simulink library "generator_lib"  (Simulink 7.8)
settings: Solver=ode45  StartTime=0.0  StopTime=10.0  RelTol=1e-3
undefined symbols (not defined in the file): dfilt, DiscIntNeverNeededParam, fdesignblkfcn, gcbh, ph, Ts
libraries: simulink x91, rtio_opalrt_common x84, powerlib x51, simulink_extras x21, discretizing x14, rteventslib x14, dsparch4 x14, powerlib_extras x4
(part 1 of 10)
settings Model: Creator=re25624  LastModifiedBy=re25624

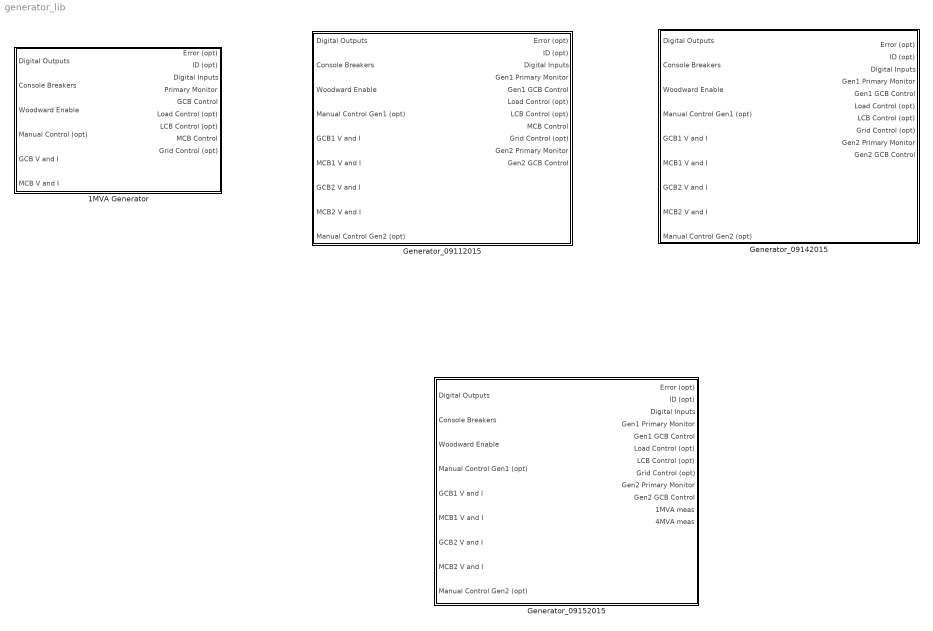
== system generator_lib ==
  1MVA Generator : Subsystem  mask{control_mode=1}
      mask prompts: control_mode "Control Mode [0 => Sim. 1 => Wood.]"
  Generator_09112015 : Subsystem
  Generator_09142015 : Subsystem
  Generator_09152015 : Subsystem  mask(Woodward and modbus controlled generators){control_mode=1}
      mask prompts: control_mode "Control Mode [0 => Sim. 1 => Wood.]"
      mask help: This block contains all the necessary logic to control two generator units (1MVA@460V and 4MVA @13.8kV) via the Woodward EasyGen controller or via Modbus commands.

== system generator_lib/1MVA Generator ==
  note: Op_Mode:
      | 0 = Relay Functions
      | 1 = Close Breaker
      | 2 = Open Breaker
  note: The woodward is set to VF mode the entire time.
  Digital Outputs : Inport
  Console Breakers : Inport  Port=2
  Woodward Enable : Inport  Port=3
  Manual Control (opt) : Inport  Port=4
  GCB V and I : Inport  Port=5
  MCB V and I : Inport  Port=6
  Bus Selector1 : BusSelector  OutputSignals=Vabc_line,Iabc
  Bus Selector5 : BusSelector  OutputSignals=Wood_DIO,Gen_bias_enable,Gen_enable,GCB,Load,LCB,Wood_MCB_enable,MCB,Grid
  Bus Selector6 : BusSelector  OutputSignals=Vabc_bus,Iabc
  Bus Selector7 : BusSelector  OutputSignals="w.w.Rotor speed  wm (pu)"
  GenSet_900kW_07232015 : Subsystem  mask(Gen-Set with simulated control modes){control_mode=control_mode}
      mask prompts: control_mode "Control Mode [0 => Sim. 1 => Wood.]"
      mask help:
      | This Gen-Set block allows the user to indicate the control mode of the generator. The available control modes are: (1) PQ, (2) PV, and (3) VF.
      | The input values to the block will be applied according to the selected control mode.
      | For example, if PQ mode is selected, the controller will only work based on P_ref and Q_ref ignoring values of other inputs to the block.
  Switch : Switch  Threshold=0.5
  Woodward Inputs : Subsystem
  Woodward Outputs : Subsystem
  A : PMIOPort  Port=1  Side=Right
  B : PMIOPort  Port=2  Side=Right
  C : PMIOPort  Port=3  Side=Right
  Error (opt) : Outport
  ID (opt) : Outport  Port=2
  Digital Inputs : Outport  Port=3
  Primary Monitor : Outport  Port=4
  GCB Control : Outport  Port=5
  Load Control (opt) : Outport  Port=6
  LCB Control (opt) : Outport  Port=7
  MCB Control : Outport  Port=8
  Grid Control (opt) : Outport  Port=9
  wires:
  Bus Selector1/2 -> Woodward Inputs/5(Mains_Current)  "<Iabc>"
  Bus Selector1/1 -> Woodward Inputs/4(Mains_Voltage)  "<Vabc_line>"
  MCB V and I/1 -> Bus Selector1/1
  Bus Selector5/9 -> Grid Control (opt)/1  "<Grid>"
  Switch/1 -> MCB Control/1
  Bus Selector5/6 -> LCB Control (opt)/1  "<LCB>"
  Bus Selector5/5 -> Load Control (opt)/1  "<Load>"
  Console Breakers/1 -> Bus Selector5/1
  Woodward Outputs/9(GCB) -> GCB Control/1
  GCB V and I/1 -> Bus Selector6/1
  Digital Outputs/1 -> Woodward Outputs/1(Digital Output)
  Woodward Outputs/10(MCB) -> Switch/1
  Bus Selector5/8 -> Switch/3  "<MCB>"
  Bus Selector5/7 -> Switch/2  "<Wood_MCB_enable>"
  Woodward Outputs/8(Fuel Enable) -> GenSet_900kW_07232015/5(Generator Enable)
  Woodward Enable/1 -> GenSet_900kW_07232015/6(Woodward Enable)
  Woodward Outputs/3(Digital Inputs) -> Digital Inputs/1
  Woodward Outputs/2(IDs) -> ID (opt)/1
  Woodward Outputs/1(Error) -> Error (opt)/1
  Bus Selector7/1 -> Woodward Inputs/1(MPU_speed)  "<Rotor speed  wm (pu)>"
  Woodward Outputs/5(Ref AVR) -> GenSet_900kW_07232015/2(Woodward Modbus Ref for AVR)
  Woodward Outputs/4(Ref Gov) -> GenSet_900kW_07232015/1(Woodward Modbus Ref for Governor)
  Bus Selector5/2 -> Woodward Outputs/3(Bias Enable)  "<Gen_bias_enable>"
  Woodward Outputs/7(AVR) -> GenSet_900kW_07232015/4(Woodward meas V)
  Woodward Outputs/6(GOV) -> GenSet_900kW_07232015/3(Woodward meas w)
  Manual Control (opt)/1 -> GenSet_900kW_07232015/7(Manual_control)
  Bus Selector5/1 -> Woodward Outputs/2(DIO Enable)  "<Wood_DIO>"
  Bus Selector6/2 -> Woodward Inputs/3(Generator_Current)  "<Iabc>"
  Bus Selector6/1 -> Woodward Inputs/2(Generator_Voltage)  "<Vabc_bus>"
  GenSet_900kW_07232015/1(gen_primary) -> Primary Monitor/1, Bus Selector7/1
  connections:
  C/RConn1 -- GenSet_900kW_07232015/RConn3
  B/RConn1 -- GenSet_900kW_07232015/RConn2
  A/RConn1 -- GenSet_900kW_07232015/RConn1

== system generator_lib/Generator_09112015 ==
  note: Ask Kendall about the output control: MCB control (8)
  note: The woodward is set to VF mode the entire time.
  note: Op_Mode:
      | 0 = Relay Functions
      | 1 = Close Breaker
      | 2 = Open Breaker
  note: Gen1: 1MVA at 460V
      | Gen2: 4MVA at 13kV
  Digital Outputs : Inport
  Console Breakers : Inport  Port=2
  Woodward Enable : Inport  Port=3
  Manual Control Gen1 (opt) : Inport  Port=4
  GCB1 V and I : Inport  Port=5
  MCB1 V and I : Inport  Port=6
  GCB2 V and I : Inport  Port=7
  MCB2 V and I : Inport  Port=8
  Manual Control Gen2 (opt) : Inport  Port=9
  Bus Selector : BusSelector  OutputSignals=Gen1 Ref GOV,Gen1 Ref AVR,Gen1 Gov,Gen1 AVR
  Bus Selector1 : BusSelector  OutputSignals=Vabc_bus,Iabc
  Bus Selector2 : BusSelector  OutputSignals="w.w.Rotor speed  wm (pu)"
  Bus Selector3 : BusSelector  OutputSignals=Vabc_line,Iabc
  Bus Selector4 : BusSelector  OutputSignals=Vabc_bus,Iabc
  Bus Selector5 : BusSelector  OutputSignals=Wood_DIO,Gen_bias_enable,Gen2_enable,Gen2_GCB,Load,LCB,Wood_MCB_enable,MCB,Grid
  Bus Selector6 : BusSelector  OutputSignals=Vabc_line,Iabc
  Bus Selector7 : BusSelector  OutputSignals="w.w.Rotor speed  wm (pu)"
  Bus Selector8 : BusSelector  OutputSignals=Gen2 Ref GOV,Gen2 Ref AVR,Gen2 GOV,Gen2 AVR
  GenSet_1MVA_09082015 : Subsystem  mask(Gen-Set with simulated control modes){control_mode=1}
      mask prompts: control_mode "Control Mode [0 => Sim. 1 => Wood.]"
      mask help:
      | This Gen-Set block allows the user to indicate the control mode of the generator. The available control modes are: (1) PQ, (2) PV, and (3) VF.
      | The input values to the block will be applied according to the selected control mode.
      | For example, if PQ mode is selected, the controller will only work based on P_ref and Q_ref ignoring values of other inputs to the block.
  GenSet_4MVA_copy1mva : Subsystem  mask(Gen-Set with simulated control modes){control_mode=1}
      mask prompts: control_mode "Control Mode [0 => Sim. 1 => Wood.]"
      mask help:
      | This Gen-Set block allows the user to indicate the control mode of the generator. The available control modes are: (1) PQ, (2) PV, and (3) VF.
      | The input values to the block will be applied according to the selected control mode.
      | For example, if PQ mode is selected, the controller will only work based on P_ref and Q_ref ignoring values of other inputs to the block.
  Switch : Switch  Threshold=0.5
  Woodward Inputs : Subsystem
  Woodward Outputs : Subsystem
  Gen2 A : PMIOPort  Port=1  Side=Right
  Gen2 B : PMIOPort  Port=2  Side=Right
  Gen2 C : PMIOPort  Port=3  Side=Right
  Gen1 A : PMIOPort  Port=4  Side=Right
  Gen1 B : PMIOPort  Port=5  Side=Right
  Gen1 C : PMIOPort  Port=6  Side=Right
  Error (opt) : Outport
  ID (opt) : Outport  Port=2
  Digital Inputs : Outport  Port=3
  Gen1 Primary Monitor : Outport  Port=4
  Gen1 GCB Control : Outport  Port=5
  Load Control (opt) : Outport  Port=6
  LCB Control (opt) : Outport  Port=7
  MCB Control : Outport  Port=8
  Grid Control (opt) : Outport  Port=9
  Gen2 Primary Monitor : Outport  Port=10
  Gen2 GCB Control : Outport  Port=11
  wires:
  GenSet_1MVA_09082015/1(gen_primary) -> Bus Selector7/1, Gen1 Primary Monitor/1
  Bus Selector6/1 -> Woodward Inputs/2(Generator1_Voltage)  "<Vabc_line>"
  Bus Selector6/2 -> Woodward Inputs/3(Generator1_Current)  "<Iabc>"
  Bus Selector5/1 -> Woodward Outputs/2(DIO Enable)  "<Wood_DIO>"
  Manual Control Gen1 (opt)/1 -> GenSet_1MVA_09082015/7(Manual_control)
  Bus Selector5/2 -> Woodward Outputs/3(Bias Enable)  "<Gen_bias_enable>"
  Bus Selector7/1 -> Woodward Inputs/1(MPU1_speed)  "<Rotor speed  wm (pu)>"
  Woodward Outputs/1(Error) -> Error (opt)/1
  Woodward Outputs/2(IDs) -> ID (opt)/1
  Woodward Outputs/3(Digital Inputs) -> Digital Inputs/1
  Woodward Enable/1 -> GenSet_1MVA_09082015/6(Woodward Enable), GenSet_4MVA_copy1mva/6(Woodward Enable)
  Woodward Outputs/6(Gen1 Fuel Enable) -> GenSet_1MVA_09082015/5(Generator Enable)
  Bus Selector5/7 -> Switch/2  "<Wood_MCB_enable>"
  Bus Selector5/8 -> Switch/3  "<MCB>"
  Woodward Outputs/8(Gen1 MCB) -> Switch/1
  Digital Outputs/1 -> Woodward Outputs/1(Digital Output)
  GCB1 V and I/1 -> Bus Selector6/1
  Woodward Outputs/7(Gen1 GCB) -> Gen1 GCB Control/1
  Console Breakers/1 -> Bus Selector5/1
  Bus Selector5/5 -> Load Control (opt)/1  "<Load>"
  Bus Selector5/6 -> LCB Control (opt)/1  "<LCB>"
  Switch/1 -> MCB Control/1
  Bus Selector5/9 -> Grid Control (opt)/1  "<Grid>"
  MCB1 V and I/1 -> Bus Selector1/1
  Bus Selector1/1 -> Woodward Inputs/4(Mains1_Voltage)  "<Vabc_bus>"
  Bus Selector1/2 -> Woodward Inputs/5(Mains1_Current)  "<Iabc>"
  GCB2 V and I/1 -> Bus Selector3/1
  MCB2 V and I/1 -> Bus Selector4/1
  GenSet_4MVA_copy1mva/1(gen_primary) -> Gen2 Primary Monitor/1, Bus Selector2/1
  Bus Selector2/1 -> Woodward Inputs/6(MPU2_speed)  "<Rotor speed  wm (pu)>"
  Bus Selector3/1 -> Woodward Inputs/7(Generator2_Voltage)  "<Vabc_line>"
  Bus Selector3/2 -> Woodward Inputs/8(Generator2_Current)  "<Iabc>"
  Bus Selector4/1 -> Woodward Inputs/9(Mains2_Voltage)  "<Vabc_bus>"
  Bus Selector4/2 -> Woodward Inputs/10(Mains2_Current)  "<Iabc>"
  Woodward Outputs/4(Gen1 Gov and AVR) -> Bus Selector/1
  Bus Selector/1 -> GenSet_1MVA_09082015/1(Woodward Modbus Ref for Governor)  "<Gen1 Ref GOV>"
  Bus Selector/2 -> GenSet_1MVA_09082015/2(Woodward Modbus Ref for AVR)  "<Gen1 Ref AVR>"
  Bus Selector/3 -> GenSet_1MVA_09082015/3(Woodward meas w)  "<Gen1 Gov>"
  Bus Selector/4 -> GenSet_1MVA_09082015/4(Woodward meas V)  "<Gen1 AVR>"
  Woodward Outputs/5(Gen2 Gov and AVR) -> Bus Selector8/1
  Bus Selector8/1 -> GenSet_4MVA_copy1mva/1(Woodward Modbus Ref for Governor)  "<Gen2 Ref GOV>"
  Bus Selector8/2 -> GenSet_4MVA_copy1mva/2(Woodward Modbus Ref for AVR)  "<Gen2 Ref AVR>"
  Bus Selector8/3 -> GenSet_4MVA_copy1mva/3(Woodward meas w)  "<Gen2 GOV>"
  Bus Selector8/4 -> GenSet_4MVA_copy1mva/4(Woodward meas V)  "<Gen2 AVR>"
  Manual Control Gen2 (opt)/1 -> GenSet_4MVA_copy1mva/7(Manual_control)
  Woodward Outputs/9(Gen2 Fuel Enable) -> GenSet_4MVA_copy1mva/5(Generator Enable)
  Woodward Outputs/10(Gen2 GCB) -> Gen2 GCB Control/1
  connections:
  Gen1 A/RConn1 -- GenSet_1MVA_09082015/RConn1
  Gen1 B/RConn1 -- GenSet_1MVA_09082015/RConn2
  Gen1 C/RConn1 -- GenSet_1MVA_09082015/RConn3
  GenSet_4MVA_copy1mva/RConn1 -- Gen2 A/RConn1
  GenSet_4MVA_copy1mva/RConn2 -- Gen2 B/RConn1
  GenSet_4MVA_copy1mva/RConn3 -- Gen2 C/RConn1

== system generator_lib/Generator_09142015 ==
  note: Gen1: 1MVA generator
      | Gen2: 4MVA generator
  note: Op_Mode:
      | 0 = Relay Functions
      | 1 = Close Breaker
      | 2 = Open Breaker
  note: The woodward is set to VF mode the entire time.
  Digital Outputs : Inport
  Console Breakers : Inport  Port=2
  Woodward Enable : Inport  Port=3
  Manual Control Gen1 (opt) : Inport  Port=4
  GCB1 V and I : Inport  Port=5
  MCB1 V and I : Inport  Port=6
  GCB2 V and I : Inport  Port=7
  MCB2 V and I : Inport  Port=8
  Manual Control Gen2 (opt) : Inport  Port=9
  Add : Sum  Inputs=+-
  Bus Selector : BusSelector  OutputSignals=Gen1 Ref GOV,Gen1 Ref AVR,Gen1 Gov,Gen1 AVR
  Bus Selector1 : BusSelector  OutputSignals=Vabc_line,Iabc
  Bus Selector2 : BusSelector  OutputSignals="w.w.Rotor speed  wm (pu)"
  Bus Selector3 : BusSelector  OutputSignals=Vabc_bus,Iabc
  Bus Selector4 : BusSelector  OutputSignals=Vabc_line,Iabc
  Bus Selector5 : BusSelector  OutputSignals=Wood_DIO,Gen_bias_enable,Gen2_enable,Gen2_GCB,Load,LCB,Wood_MCB_enable,MCB,Grid
  Bus Selector6 : BusSelector  OutputSignals=Vabc_bus,Iabc
  Bus Selector7 : BusSelector  OutputSignals="w.w.Rotor speed  wm (pu)"
  Bus Selector8 : BusSelector  OutputSignals=Gen2 Ref GOV,Gen2 Ref AVR,Gen2 GOV,Gen2 AVR
  Constant : Constant  Value=0.01
  GenSet_1MVA_09082015 : Subsystem  mask(Gen-Set with simulated control modes){control_mode=1}
      mask prompts: control_mode "Control Mode [0 => Sim. 1 => Wood.]"
      mask help:
      | This Gen-Set block allows the user to indicate the control mode of the generator. The available control modes are: (1) PQ, (2) PV, and (3) VF.
      | The input values to the block will be applied according to the selected control mode.
      | For example, if PQ mode is selected, the controller will only work based on P_ref and Q_ref ignoring values of other inputs to the block.
  GenSet_4MVA_09142015 : Subsystem  mask(Gen-Set with simulated control modes){control_mode=1}
      mask prompts: control_mode "Control Mode [0 => Sim. 1 => Wood.]"
      mask help:
      | This Gen-Set block allows the user to indicate the control mode of the generator. The available control modes are: (1) PQ, (2) PV, and (3) VF.
      | The input values to the block will be applied according to the selected control mode.
      | For example, if PQ mode is selected, the controller will only work based on P_ref and Q_ref ignoring values of other inputs to the block.
  Woodward Inputs : Subsystem
  Woodward Outputs : Subsystem
  Gen2 A : PMIOPort  Port=1  Side=Right
  Gen2 B : PMIOPort  Port=2  Side=Right
  Gen2 C : PMIOPort  Port=3  Side=Right
  Gen1 A : PMIOPort  Port=4  Side=Right
  Gen1 B : PMIOPort  Port=5  Side=Right
  Gen1 C : PMIOPort  Port=6  Side=Right
  Error (opt) : Outport
  ID (opt) : Outport  Port=2
  Digital Inputs : Outport  Port=3
  Gen1 Primary Monitor : Outport  Port=4
  Gen1 GCB Control : Outport  Port=5
  Load Control (opt) : Outport  Port=6
  LCB Control (opt) : Outport  Port=7
  Grid Control (opt) : Outport  Port=8
  Gen2 Primary Monitor : Outport  Port=9
  Gen2 GCB Control : Outport  Port=10
  wires:
  Constant/1 -> Add/2
  Add/1 -> Woodward Inputs/6(MPU2_speed)
  Woodward Outputs/10(Gen2 GCB) -> Gen2 GCB Control/1
  Woodward Outputs/9(Gen2 Fuel Enable) -> GenSet_4MVA_09142015/5(Generator Enable)
  Manual Control Gen2 (opt)/1 -> GenSet_4MVA_09142015/7(Manual_control)
  Bus Selector8/4 -> GenSet_4MVA_09142015/4(Woodward meas V)  "<Gen2 AVR>"
  Bus Selector8/3 -> GenSet_4MVA_09142015/3(Woodward meas w)  "<Gen2 GOV>"
  Bus Selector8/2 -> GenSet_4MVA_09142015/2(Woodward Modbus Ref for AVR)  "<Gen2 Ref AVR>"
  Bus Selector8/1 -> GenSet_4MVA_09142015/1(Woodward Modbus Ref for Governor)  "<Gen2 Ref GOV>"
  Woodward Outputs/5(Gen2 Gov and AVR) -> Bus Selector8/1
  Bus Selector/4 -> GenSet_1MVA_09082015/4(Woodward meas V)  "<Gen1 AVR>"
  Bus Selector/3 -> GenSet_1MVA_09082015/3(Woodward meas w)  "<Gen1 Gov>"
  Bus Selector/2 -> GenSet_1MVA_09082015/2(Woodward Modbus Ref for AVR)  "<Gen1 Ref AVR>"
  Bus Selector/1 -> GenSet_1MVA_09082015/1(Woodward Modbus Ref for Governor)  "<Gen1 Ref GOV>"
  Woodward Outputs/4(Gen1 Gov and AVR) -> Bus Selector/1
  Bus Selector4/2 -> Woodward Inputs/10(Mains2_Current)  "<Iabc>"
  Bus Selector4/1 -> Woodward Inputs/9(Mains2_Voltage)  "<Vabc_line>"
  Bus Selector3/2 -> Woodward Inputs/8(Generator2_Current)  "<Iabc>"
  Bus Selector3/1 -> Woodward Inputs/7(Generator2_Voltage)  "<Vabc_bus>"
  Bus Selector2/1 -> Add/1  "<Rotor speed  wm (pu)>"
  GenSet_4MVA_09142015/1(gen_primary) -> Bus Selector2/1, Gen2 Primary Monitor/1
  MCB2 V and I/1 -> Bus Selector4/1
  GCB2 V and I/1 -> Bus Selector3/1
  Bus Selector1/2 -> Woodward Inputs/5(Mains1_Current)  "<Iabc>"
  Bus Selector1/1 -> Woodward Inputs/4(Mains1_Voltage)  "<Vabc_line>"
  MCB1 V and I/1 -> Bus Selector1/1
  Bus Selector5/9 -> Grid Control (opt)/1  "<Grid>"
  Bus Selector5/6 -> LCB Control (opt)/1  "<LCB>"
  Bus Selector5/5 -> Load Control (opt)/1  "<Load>"
  Console Breakers/1 -> Bus Selector5/1
  Woodward Outputs/7(Gen1 GCB) -> Gen1 GCB Control/1
  GCB1 V and I/1 -> Bus Selector6/1
  Digital Outputs/1 -> Woodward Outputs/1(Digital Output)
  Woodward Outputs/6(Gen1 Fuel Enable) -> GenSet_1MVA_09082015/5(Generator Enable)
  Woodward Enable/1 -> GenSet_4MVA_09142015/6(Woodward Enable), GenSet_1MVA_09082015/6(Woodward Enable)
  Woodward Outputs/3(Digital Inputs) -> Digital Inputs/1
  Woodward Outputs/2(IDs) -> ID (opt)/1
  Woodward Outputs/1(Error) -> Error (opt)/1
  Bus Selector7/1 -> Woodward Inputs/1(MPU1_speed)  "<Rotor speed  wm (pu)>"
  Bus Selector5/2 -> Woodward Outputs/3(Bias Enable)  "<Gen_bias_enable>"
  Manual Control Gen1 (opt)/1 -> GenSet_1MVA_09082015/7(Manual_control)
  Bus Selector5/1 -> Woodward Outputs/2(DIO Enable)  "<Wood_DIO>"
  Bus Selector6/2 -> Woodward Inputs/3(Generator1_Current)  "<Iabc>"
  Bus Selector6/1 -> Woodward Inputs/2(Generator1_Voltage)  "<Vabc_bus>"
  GenSet_1MVA_09082015/1(gen_primary) -> Gen1 Primary Monitor/1, Bus Selector7/1
  connections:
  GenSet_4MVA_09142015/RConn3 -- Gen2 C/RConn1
  GenSet_4MVA_09142015/RConn2 -- Gen2 B/RConn1
  GenSet_4MVA_09142015/RConn1 -- Gen2 A/RConn1
  Gen1 C/RConn1 -- GenSet_1MVA_09082015/RConn3
  Gen1 B/RConn1 -- GenSet_1MVA_09082015/RConn2
  Gen1 A/RConn1 -- GenSet_1MVA_09082015/RConn1

== system generator_lib/Generator_09152015 ==
  note: Gen1: 1MVA generator
      | Gen2: 4MVA generator
  note: Op_Mode:
      | 0 = Relay Functions
      | 1 = Close Breaker
      | 2 = Open Breaker
  note: The woodward is set to VF mode the entire time.
  note: When used in the system to be simulated,
      | this model most be disabled from the library or the I/Os will have an error
  Digital Outputs : Inport
  Console Breakers : Inport  Port=2
  Woodward Enable : Inport  Port=3
  Manual Control Gen1 (opt) : Inport  Port=4
  GCB1 V and I : Inport  Port=5
  MCB1 V and I : Inport  Port=6
  GCB2 V and I : Inport  Port=7
  MCB2 V and I : Inport  Port=8
  Manual Control Gen2 (opt) : Inport  Port=9
  Add : Sum  Inputs=+-
  Bus Selector : BusSelector  OutputSignals=Gen1 Ref GOV,Gen1 Ref AVR,Gen1 Gov,Gen1 AVR
  Bus Selector1 : BusSelector  OutputSignals=Vabc_line,Iabc
  Bus Selector2 : BusSelector  OutputSignals="w.w.Rotor speed  wm (pu)"
  Bus Selector3 : BusSelector  OutputSignals=Vabc_bus,Iabc
  Bus Selector4 : BusSelector  OutputSignals=Vabc_line,Iabc
  Bus Selector5 : BusSelector  OutputSignals=Wood_DIO,Gen_bias_enable,Gen2_enable,Gen2_GCB,Load,LCB,Wood_MCB_enable,MCB,Grid
  Bus Selector6 : BusSelector  OutputSignals=Vabc_bus,Iabc
  Bus Selector7 : BusSelector  OutputSignals="w.w.Rotor speed  wm (pu)"
  Bus Selector8 : BusSelector  OutputSignals=Gen2 Ref GOV,Gen2 Ref AVR,Gen2 GOV,Gen2 AVR
  Constant : Constant  Value=0.01
  GenSet_1MVA_09082015 : Subsystem  mask(Gen-Set with simulated control modes){control_mode=control_mode}
      mask prompts: control_mode "Control Mode [0 => Sim. 1 => Wood.]"
      mask help:
      | This Gen-Set block allows the user to indicate the control mode of the generator. The available control modes are: (1) PQ, (2) PV, and (3) VF.
      | The input values to the block will be applied according to the selected control mode.
      | For example, if PQ mode is selected, the controller will only work based on P_ref and Q_ref ignoring values of other inputs to the block.
  GenSet_4MVA_09142015 : Subsystem  mask(Gen-Set with simulated control modes){control_mode=control_mode}
      mask prompts: control_mode "Control Mode [0 => Sim. 1 => Wood.]"
      mask help:
      | This Gen-Set block allows the user to indicate the control mode of the generator. The available control modes are: (1) PQ, (2) PV, and (3) VF.
      | The input values to the block will be applied according to the selected control mode.
      | For example, if PQ mode is selected, the controller will only work based on P_ref and Q_ref ignoring values of other inputs to the block.
  Woodward Inputs : Subsystem
  Woodward Outputs : Subsystem
  Gen2 A : PMIOPort  Port=1  Side=Right
  Gen2 B : PMIOPort  Port=2  Side=Right
  Gen2 C : PMIOPort  Port=3  Side=Right
  Gen1 A : PMIOPort  Port=4  Side=Right
  Gen1 B : PMIOPort  Port=5  Side=Right
  Gen1 C : PMIOPort  Port=6  Side=Right
  Error (opt) : Outport
  ID (opt) : Outport  Port=2
  Digital Inputs : Outport  Port=3
  Gen1 Primary Monitor : Outport  Port=4
  Gen1 GCB Control : Outport  Port=5
  Load Control (opt) : Outport  Port=6
  LCB Control (opt) : Outport  Port=7
  Grid Control (opt) : Outport  Port=8
  Gen2 Primary Monitor : Outport  Port=9
  Gen2 GCB Control : Outport  Port=10
  1MVA meas : Outport  Port=11
  4MVA meas : Outport  Port=12
  wires:
  GenSet_4MVA_09142015/2(gen_output) -> 4MVA meas/1
  GenSet_1MVA_09082015/2(gen_output) -> 1MVA meas/1
  Constant/1 -> Add/2
  Add/1 -> Woodward Inputs/6(MPU2_speed)
  Woodward Outputs/10(Gen2 GCB) -> Gen2 GCB Control/1
  Woodward Outputs/9(Gen2 Fuel Enable) -> GenSet_4MVA_09142015/5(Generator Enable)
  Manual Control Gen2 (opt)/1 -> GenSet_4MVA_09142015/7(Manual_control)
  Bus Selector8/4 -> GenSet_4MVA_09142015/4(Woodward meas V)  "<Gen2 AVR>"
  Bus Selector8/3 -> GenSet_4MVA_09142015/3(Woodward meas w)  "<Gen2 GOV>"
  Bus Selector8/2 -> GenSet_4MVA_09142015/2(Woodward Modbus Ref for AVR)  "<Gen2 Ref AVR>"
  Bus Selector8/1 -> GenSet_4MVA_09142015/1(Woodward Modbus Ref for Governor)  "<Gen2 Ref GOV>"
  Woodward Outputs/5(Gen2 Gov and AVR) -> Bus Selector8/1
  Bus Selector/4 -> GenSet_1MVA_09082015/4(Woodward meas V)  "<Gen1 AVR>"
  Bus Selector/3 -> GenSet_1MVA_09082015/3(Woodward meas w)  "<Gen1 Gov>"
  Bus Selector/2 -> GenSet_1MVA_09082015/2(Woodward Modbus Ref for AVR)  "<Gen1 Ref AVR>"
  Bus Selector/1 -> GenSet_1MVA_09082015/1(Woodward Modbus Ref for Governor)  "<Gen1 Ref GOV>"
  Woodward Outputs/4(Gen1 Gov and AVR) -> Bus Selector/1
  Bus Selector4/2 -> Woodward Inputs/10(Mains2_Current)  "<Iabc>"
  Bus Selector4/1 -> Woodward Inputs/9(Mains2_Voltage)  "<Vabc_line>"
  Bus Selector3/2 -> Woodward Inputs/8(Generator2_Current)  "<Iabc>"
  Bus Selector3/1 -> Woodward Inputs/7(Generator2_Voltage)  "<Vabc_bus>"
  Bus Selector2/1 -> Add/1  "<Rotor speed  wm (pu)>"
  GenSet_4MVA_09142015/1(gen_primary) -> Bus Selector2/1, Gen2 Primary Monitor/1
  MCB2 V and I/1 -> Bus Selector4/1
  GCB2 V and I/1 -> Bus Selector3/1
  Bus Selector1/2 -> Woodward Inputs/5(Mains1_Current)  "<Iabc>"
  Bus Selector1/1 -> Woodward Inputs/4(Mains1_Voltage)  "<Vabc_line>"
  MCB1 V and I/1 -> Bus Selector1/1
  Bus Selector5/9 -> Grid Control (opt)/1  "<Grid>"
  Bus Selector5/6 -> LCB Control (opt)/1  "<LCB>"
  Bus Selector5/5 -> Load Control (opt)/1  "<Load>"
  Console Breakers/1 -> Bus Selector5/1
  Woodward Outputs/7(Gen1 GCB) -> Gen1 GCB Control/1
  GCB1 V and I/1 -> Bus Selector6/1
  Digital Outputs/1 -> Woodward Outputs/1(Digital Output)
  Woodward Outputs/6(Gen1 Fuel Enable) -> GenSet_1MVA_09082015/5(Generator Enable)
  Woodward Enable/1 -> GenSet_4MVA_09142015/6(Woodward Enable), GenSet_1MVA_09082015/6(Woodward Enable)
  Woodward Outputs/3(Digital Inputs) -> Digital Inputs/1
  Woodward Outputs/2(IDs) -> ID (opt)/1
  Woodward Outputs/1(Error) -> Error (opt)/1
  Bus Selector7/1 -> Woodward Inputs/1(MPU1_speed)  "<Rotor speed  wm (pu)>"
  Bus Selector5/2 -> Woodward Outputs/3(Bias Enable)  "<Gen_bias_enable>"
  Manual Control Gen1 (opt)/1 -> GenSet_1MVA_09082015/7(Manual_control)
  Bus Selector5/1 -> Woodward Outputs/2(DIO Enable)  "<Wood_DIO>"
  Bus Selector6/2 -> Woodward Inputs/3(Generator1_Current)  "<Iabc>"
  Bus Selector6/1 -> Woodward Inputs/2(Generator1_Voltage)  "<Vabc_bus>"
  GenSet_1MVA_09082015/1(gen_primary) -> Gen1 Primary Monitor/1, Bus Selector7/1
  connections:
  GenSet_4MVA_09142015/RConn3 -- Gen2 C/RConn1
  GenSet_4MVA_09142015/RConn2 -- Gen2 B/RConn1
  GenSet_4MVA_09142015/RConn1 -- Gen2 A/RConn1
  Gen1 C/RConn1 -- GenSet_1MVA_09082015/RConn3
  Gen1 B/RConn1 -- GenSet_1MVA_09082015/RConn2
  Gen1 A/RConn1 -- GenSet_1MVA_09082015/RConn1

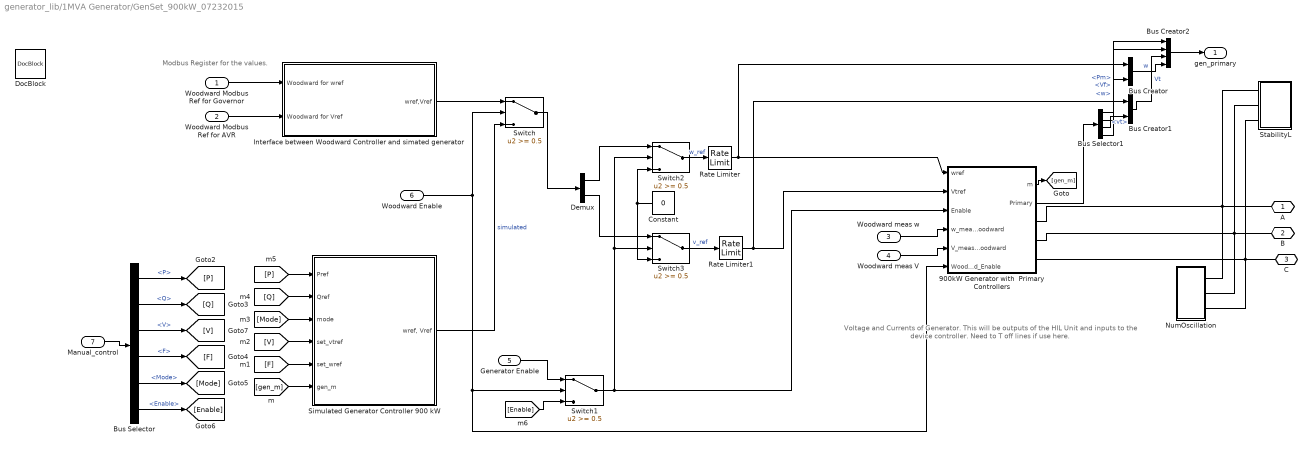
== system generator_lib/1MVA Generator/GenSet_900kW_07232015 ==
  note: Voltage and Currents of Generator.
      | This will be outputs of the HIL Unit
      | and inputs to the device controller.
      | Need to T off lines if use here.
  note: Modbus Register for the values.
  Woodward Modbus Ref for Governor : Inport
  Woodward Modbus Ref for AVR : Inport  Port=2
  Woodward meas w : Inport  Port=3
  Woodward meas V : Inport  Port=4
  Generator Enable : Inport  Port=5
  Woodward Enable : Inport  Port=6
  Manual_control : Inport  Port=7
  900kW Generator with  Primary Controllers : Subsystem
  Bus Creator : BusCreator  Inputs=2
  Bus Creator1 : BusCreator  Inputs=2
  Bus Creator2 : BusCreator
  Bus Selector : BusSelector  OutputSignals=P,Q,V,F,Mode,Enable
  Bus Selector1 : BusSelector  OutputSignals=Pm,Vf,vt,w
  Constant : Constant  Value=0
  Demux : Demux  Outputs=2
  DocBlock : simulink/Model-Wide Utilities/DocBlock  DocumentType=Text
  Interface between Woodward Controller and simated generator : Subsystem
  NumOscillation : Subsystem
  Rate Limiter : RateLimiter  RisingSlewLimit=0.5  FallingSlewLimit=-0.5  SampleTimeMode=inherited
  Rate Limiter1 : RateLimiter  RisingSlewLimit=0.5  FallingSlewLimit=-0.5  SampleTimeMode=inherited
  Simulated Generator Controller 900 kW : Subsystem
  StabilityL : Subsystem  mask{v=460, kVA=50, pf=1}
  Switch{,1..3} (4 alike) : Switch  Threshold=0.5
  A : PMIOPort  Port=1  Side=Right
  B : PMIOPort  Port=2  Side=Right
  C : PMIOPort  Port=3  Side=Right
  gen_primary : Outport
  wires:
  Woodward Enable/1 -> 900kW Generator with  Primary Controllers/6(Woodward_Enable), Switch1/2, Switch/2
  Rate Limiter1/1 -> Bus Creator1/1, 900kW Generator with  Primary Controllers/2(Vtref)
  Rate Limiter/1 -> Bus Creator/1, 900kW Generator with  Primary Controllers/1(wref)
  Bus Creator2/1 -> gen_primary/1
  Bus Creator/1 -> Bus Creator2/4  "w"
  Bus Creator1/1 -> Bus Creator2/3  "Vt"
  Bus Selector1/1 -> Bus Creator2/1  "<Pm>"
  Bus Selector1/2 -> Bus Creator2/2  "<Vf>"
  Bus Selector1/4 -> Bus Creator/2  "<w>"
  Bus Selector1/3 -> Bus Creator1/2  "<vt>"
  Switch3/1 -> Rate Limiter1/1  "v_ref"
  Constant/1 -> Switch2/3, Switch3/3
  Demux/2 -> Switch3/1
  Demux/1 -> Switch2/1
  Switch2/1 -> Rate Limiter/1  "w_ref"
  Switch1/1 -> Switch3/2, Switch2/2, 900kW Generator with  Primary Controllers/3(Enable)
  [Enable] -> Switch1/3
  Generator Enable/1 -> Switch1/1
  900kW Generator with  Primary Controllers/2(Primary) -> Bus Selector1/1
  Bus Selector/6 -> [Enable]  "<Enable>"
  Woodward meas V/1 -> 900kW Generator with  Primary Controllers/5(V_meas_Woodward)
  Woodward meas w/1 -> 900kW Generator with  Primary Controllers/4(w_meas_Woodward)
  Woodward Modbus Ref for AVR/1 -> Interface between Woodward Controller and simated generator/2(Woodward for Vref)
  Woodward Modbus Ref for Governor/1 -> Interface between Woodward Controller and simated generator/1(Woodward for wref)
  Switch/1 -> Demux/1
  Interface between Woodward Controller and simated generator/1(wref,Vref) -> Switch/1
  900kW Generator with  Primary Controllers/1(m) -> [gen_m]
  Simulated Generator Controller 900 kW/1("wref, Vref") -> Switch/3  "simulated"
  Manual_control/1 -> Bus Selector/1
  Bus Selector/1 -> [P]  "<P>"
  Bus Selector/2 -> [Q]  "<Q>"
  Bus Selector/3 -> [V]  "<V>"
  Bus Selector/4 -> [F]  "<F>"
  Bus Selector/5 -> [Mode]  "<Mode>"
  [gen_m] -> Simulated Generator Controller 900 kW/6(gen_m)
  [P] -> Simulated Generator Controller 900 kW/1(Pref)
  [Q] -> Simulated Generator Controller 900 kW/2(Qref)
  [Mode] -> Simulated Generator Controller 900 kW/3(mode)
  [V] -> Simulated Generator Controller 900 kW/4(set_vtref)
  [F] -> Simulated Generator Controller 900 kW/5(set_wref)
  connections:
  NumOscillation/LConn3 -- 900kW Generator with  Primary Controllers/RConn3 -- C/RConn1 -- StabilityL/LConn3
  NumOscillation/LConn2 -- B/RConn1 -- 900kW Generator with  Primary Controllers/RConn2 -- StabilityL/LConn2
  NumOscillation/LConn1 -- 900kW Generator with  Primary Controllers/RConn1 -- A/RConn1 -- StabilityL/LConn1

== system generator_lib/1MVA Generator/Woodward Inputs ==
  note: Wood 3.5MW 3/P
      | Mains Voltage
  note: Wood 3.5MW 3/P
      | Gen. Voltage
  note: Wood 3.5MW MPU
  note: There will need to be a
      | new scaling factor to use
      | the current cards (0-1A)
  note: GR1 A AOUT (CH00-15)
  note: For 120 => 12Vout / 170Vpk
      | For 480 => 12Vout / 391Vpk
      | For 13.8kv => 12Vout / 11268Vpk
  note: 6Vout / ( 900,000W / 391 Vpk)
  MPU_speed : Inport
  Generator_Voltage : Inport  Port=2
  Generator_Current : Inport  Port=3
  Mains_Voltage : Inport  Port=4
  Mains_Current : Inport  Port=5
  AnalogOut : rtio_opalrt_common/AnalogOut  CtrlName='OpCtrl'  portNb=1  FcnNos=Slot 1 Module A Subsection 1  size=16  maxcount=-2  count=8  numchan=8  israngeinput=off  voltagerange=[-16 ... 16]  slot=0  side=0  mismatch=0  slotside=Slot_1_Module_A
      settings: AttributesFormatString=%<CtrlName>
  AnalogOut1 : rtio_opalrt_common/AnalogOut  CtrlName='OpCtrl'  portNb=2  FcnNos=Slot 1 Module A Subsection 2  size=16  maxcount=-2  count=8  numchan=8  israngeinput=off  voltagerange=[-16 ... 16]  slot=0  side=0  mismatch=0  slotside=Slot_1_Module_A
      settings: AttributesFormatString=%<CtrlName>
  AnalogOut2 : rtio_opalrt_common/AnalogOut  CtrlName='OpCtrl'  portNb=3  FcnNos=Slot 2 Module A Subsection 1  size=16  maxcount=-2  count=8  numchan=8  israngeinput=off  voltagerange=[-16 ... 16]  slot=1  side=0  mismatch=0  slotside=Slot_2_Module_A
      settings: AttributesFormatString=%<CtrlName>
  AnalogOut3 : rtio_opalrt_common/AnalogOut  CtrlName='OpCtrl'  portNb=4  FcnNos=Slot 2 Module A Subsection 2  size=16  maxcount=-2  count=8  numchan=8  israngeinput=off  voltagerange=[-16 ... 16]  slot=1  side=0  mismatch=0  slotside=Slot_2_Module_A
      settings: AttributesFormatString=%<CtrlName>
  Demux : Demux  Outputs=2
  Demux{1..5,7} (6 alike) : Demux  Outputs=3
  Demux6 : Demux  Outputs=2
  Gain : Gain  Gain=15/391
  Gain1 : Gain  Gain=15/11268
  Gain2 : Gain  Gain=15/(900000/391)
  Gain3 : Gain  Gain=15/(900000/11268)
  Mux{,1,3..4} (4 alike) : Mux  Inputs=8
  Mux2 : Mux  Inputs=2
  Mux5 : Mux  Inputs=2
  Speed_System : Subsystem
  Terminator{,1..3} (4 alike) : Terminator
  wires:
  Demux7/1 -> Mux3/1
  Gain3/1 -> Demux7/1
  Mains_Current/1 -> Gain3/1
  Demux3/3 -> Mux3/4
  Demux3/2 -> Mux3/3
  Demux3/1 -> Mux3/2
  Gain2/1 -> Demux3/1
  AnalogOut2/1 -> Terminator2/1
  AnalogOut3/1 -> Terminator3/1
  Demux6/1 -> AnalogOut2/1
  Demux6/2 -> AnalogOut3/1
  Mux3/1 -> Mux5/1
  Mux4/1 -> Mux5/2
  Mux5/1 -> Demux6/1
  Demux5/3 -> Mux1/4
  Demux5/2 -> Mux1/3
  Demux5/1 -> Mux1/2
  Demux4/3 -> Mux1/1
  Demux4/2 -> Mux/8
  Demux4/1 -> Mux/7
  Speed_System/1(Out1) -> Mux1/5
  Demux2/3 -> Mux/6
  Demux2/2 -> Mux/5
  Demux2/1 -> Mux/4
  Demux1/3 -> Mux/3
  Demux1/2 -> Mux/2
  Demux1/1 -> Mux/1
  AnalogOut/1 -> Terminator/1
  AnalogOut1/1 -> Terminator1/1
  Demux/1 -> AnalogOut/1
  Demux/2 -> AnalogOut1/1
  Generator_Voltage/1 -> Gain/1
  Mux/1 -> Mux2/1
  Mux1/1 -> Mux2/2
  Mux2/1 -> Demux/1
  Mains_Voltage/1 -> Gain1/1
  Gain/1 -> Demux1/1
  Gain1/1 -> Demux2/1
  Generator_Current/1 -> Gain2/1
  MPU_speed/1 -> Speed_System/1(In1)

== system generator_lib/1MVA Generator/Woodward Outputs ==
  Digital Output : Inport
  DIO Enable : Inport  Port=2
  Bias Enable : Inport  Port=3
  Bus Creator1 : BusCreator  Inputs=3
  Bus Selector : BusSelector  OutputSignals=DIN.DI_CH00-07.Starter,DIN.DI_CH00-07.Fuel_Solenoid
  Compare To Zero : simulink/Logic and Bit Operations/Compare To Zero  relop=>  OutDataTypeStr=boolean
  Compare To Zero1 : simulink/Logic and Bit Operations/Compare To Zero  relop=<=  OutDataTypeStr=boolean
  Constant : Constant
  Constant1 : Constant  Value=0
  DIO - Gr3 : Subsystem
  DIO - Woodward : Subsystem
  DOUT type config : Subsystem
  OpCtrl : rtio_opalrt_common/OpCtrl  CtrlName='OpCtrl'  boardid=0  BitstreamFilename=VC707_2-EX-0001-2_2_6_61-32AIO16DIO16DIOSel-01-01.bin  numconfig=-1  mode=Master  externalClock=off  decimRtsi=0  calibIO=off  SampleTime=0  loadinport=-1  BoardType=VC707  SecondaryPresent=off  sync_type=Audio
  PWM IO - Gr3 : Subsystem
  S-R Flip-Flop : simulink_extras/Flip Flops/S-R Flip-Flop  initial_condition=0
  Switch : Switch  Threshold=0.5
  TSDIO - Gr3 : Subsystem
  Woodward Primary Inputs : Subsystem
  Error : Outport
  IDs : Outport  Port=2
  Digital Inputs : Outport  Port=3
  Ref Gov : Outport  Port=4
  Ref AVR : Outport  Port=5
  GOV : Outport  Port=6
  AVR : Outport  Port=7
  Fuel Enable : Outport  Port=8
  GCB : Outport  Port=9
  MCB : Outport  Port=10
  wires:
  DIO - Woodward/2(MCB) -> MCB/1
  DIO - Woodward/1(GCB) -> GCB/1
  Compare To Zero1/1 -> S-R Flip-Flop/2
  Switch/1 -> Fuel Enable/1
  Constant/1 -> Switch/1
  Constant1/1 -> Switch/3
  Compare To Zero/1 -> S-R Flip-Flop/1
  S-R Flip-Flop/1 -> Switch/2
  Bus Selector/2 -> Compare To Zero1/1  "<Fuel_Solenoid>"
  Bus Selector/1 -> Compare To Zero/1  "<Starter>"
  Digital Output/1 -> TSDIO - Gr3/1(TSDout), PWM IO - Gr3/1(PWMOut), DIO - Woodward/2(Din_sim)
  Woodward Primary Inputs/4(AVR) -> AVR/1
  Woodward Primary Inputs/3(GOV) -> GOV/1
  Bias Enable/1 -> Woodward Primary Inputs/1(Bias-ctrl)
  Woodward Primary Inputs/2(Ref AVR) -> Ref AVR/1
  Woodward Primary Inputs/1(Ref Gov) -> Ref Gov/1
  DIO Enable/1 -> DIO - Woodward/3(control)
  Bus Creator1/1 -> Bus Selector/1, Digital Inputs/1
  DIO - Gr3/1(DIn) -> DIO - Woodward/1(Din_wood), Bus Creator1/1  "DIN"
  TSDIO - Gr3/1(TSDin) -> Bus Creator1/2  "TSDIN"
  PWM IO - Gr3/1(PWMIn) -> Bus Creator1/3  "PWMIN"
  DIO - Woodward/3(DIn) -> DIO - Gr3/1(Dout)
  OpCtrl/2 -> IDs/1
  OpCtrl/1 -> Error/1

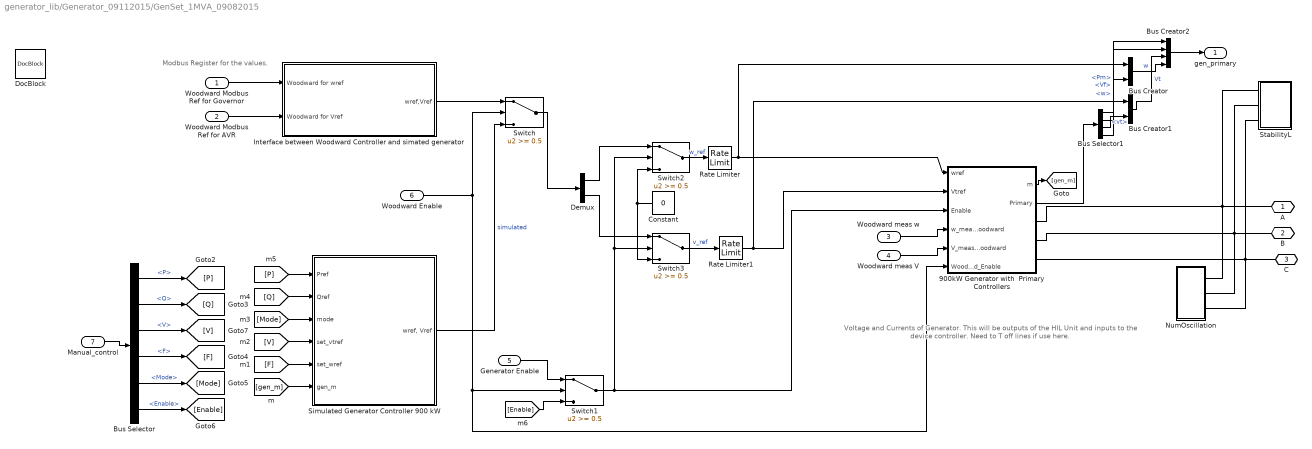
== system generator_lib/Generator_09112015/GenSet_1MVA_09082015 ==
  note: Modbus Register for the values.
  note: Voltage and Currents of Generator.
      | This will be outputs of the HIL Unit
      | and inputs to the device controller.
      | Need to T off lines if use here.
  Woodward Modbus Ref for Governor : Inport
  Woodward Modbus Ref for AVR : Inport  Port=2
  Woodward meas w : Inport  Port=3
  Woodward meas V : Inport  Port=4
  Generator Enable : Inport  Port=5
  Woodward Enable : Inport  Port=6
  Manual_control : Inport  Port=7
  900kW Generator with  Primary Controllers : Subsystem
  Bus Creator : BusCreator  Inputs=2
  Bus Creator1 : BusCreator  Inputs=2
  Bus Creator2 : BusCreator
  Bus Selector : BusSelector  OutputSignals=P,Q,V,F,Mode,Enable
  Bus Selector1 : BusSelector  OutputSignals=Pm,Vf,vt,w
  Constant : Constant  Value=0
  Demux : Demux  Outputs=2
  DocBlock : simulink/Model-Wide Utilities/DocBlock  DocumentType=Text
  Interface between Woodward Controller and simated generator : Subsystem
  NumOscillation : Subsystem
  Rate Limiter : RateLimiter  RisingSlewLimit=0.5  FallingSlewLimit=-0.5  SampleTimeMode=inherited
  Rate Limiter1 : RateLimiter  RisingSlewLimit=0.5  FallingSlewLimit=-0.5  SampleTimeMode=inherited
  Simulated Generator Controller 900 kW : Subsystem
  StabilityL : Subsystem  mask{v=460, kVA=50, pf=1}
  Switch{,1..3} (4 alike) : Switch  Threshold=0.5
  A : PMIOPort  Port=1  Side=Right
  B : PMIOPort  Port=2  Side=Right
  C : PMIOPort  Port=3  Side=Right
  gen_primary : Outport
  wires:
  [F] -> Simulated Generator Controller 900 kW/5(set_wref)
  [V] -> Simulated Generator Controller 900 kW/4(set_vtref)
  [Mode] -> Simulated Generator Controller 900 kW/3(mode)
  [Q] -> Simulated Generator Controller 900 kW/2(Qref)
  [P] -> Simulated Generator Controller 900 kW/1(Pref)
  [gen_m] -> Simulated Generator Controller 900 kW/6(gen_m)
  Bus Selector/5 -> [Mode]  "<Mode>"
  Bus Selector/4 -> [F]  "<F>"
  Bus Selector/3 -> [V]  "<V>"
  Bus Selector/2 -> [Q]  "<Q>"
  Bus Selector/1 -> [P]  "<P>"
  Manual_control/1 -> Bus Selector/1
  Simulated Generator Controller 900 kW/1("wref, Vref") -> Switch/3  "simulated"
  900kW Generator with  Primary Controllers/1(m) -> [gen_m]
  Interface between Woodward Controller and simated generator/1(wref,Vref) -> Switch/1
  Switch/1 -> Demux/1
  Woodward Modbus Ref for Governor/1 -> Interface between Woodward Controller and simated generator/1(Woodward for wref)
  Woodward Modbus Ref for AVR/1 -> Interface between Woodward Controller and simated generator/2(Woodward for Vref)
  Woodward meas w/1 -> 900kW Generator with  Primary Controllers/4(w_meas_Woodward)
  Woodward meas V/1 -> 900kW Generator with  Primary Controllers/5(V_meas_Woodward)
  Bus Selector/6 -> [Enable]  "<Enable>"
  900kW Generator with  Primary Controllers/2(Primary) -> Bus Selector1/1
  Generator Enable/1 -> Switch1/1
  [Enable] -> Switch1/3
  Switch1/1 -> 900kW Generator with  Primary Controllers/3(Enable), Switch2/2, Switch3/2
  Switch2/1 -> Rate Limiter/1  "w_ref"
  Demux/1 -> Switch2/1
  Demux/2 -> Switch3/1
  Constant/1 -> Switch3/3, Switch2/3
  Switch3/1 -> Rate Limiter1/1  "v_ref"
  Bus Selector1/3 -> Bus Creator1/2  "<vt>"
  Bus Selector1/4 -> Bus Creator/2  "<w>"
  Bus Selector1/2 -> Bus Creator2/2  "<Vf>"
  Bus Selector1/1 -> Bus Creator2/1  "<Pm>"
  Bus Creator1/1 -> Bus Creator2/3  "Vt"
  Bus Creator/1 -> Bus Creator2/4  "w"
  Bus Creator2/1 -> gen_primary/1
  Rate Limiter/1 -> 900kW Generator with  Primary Controllers/1(wref), Bus Creator/1
  Rate Limiter1/1 -> 900kW Generator with  Primary Controllers/2(Vtref), Bus Creator1/1
  Woodward Enable/1 -> Switch/2, Switch1/2, 900kW Generator with  Primary Controllers/6(Woodward_Enable)
  connections:
  StabilityL/LConn1 -- A/RConn1 -- 900kW Generator with  Primary Controllers/RConn1 -- NumOscillation/LConn1
  StabilityL/LConn2 -- 900kW Generator with  Primary Controllers/RConn2 -- B/RConn1 -- NumOscillation/LConn2
  StabilityL/LConn3 -- C/RConn1 -- 900kW Generator with  Primary Controllers/RConn3 -- NumOscillation/LConn3

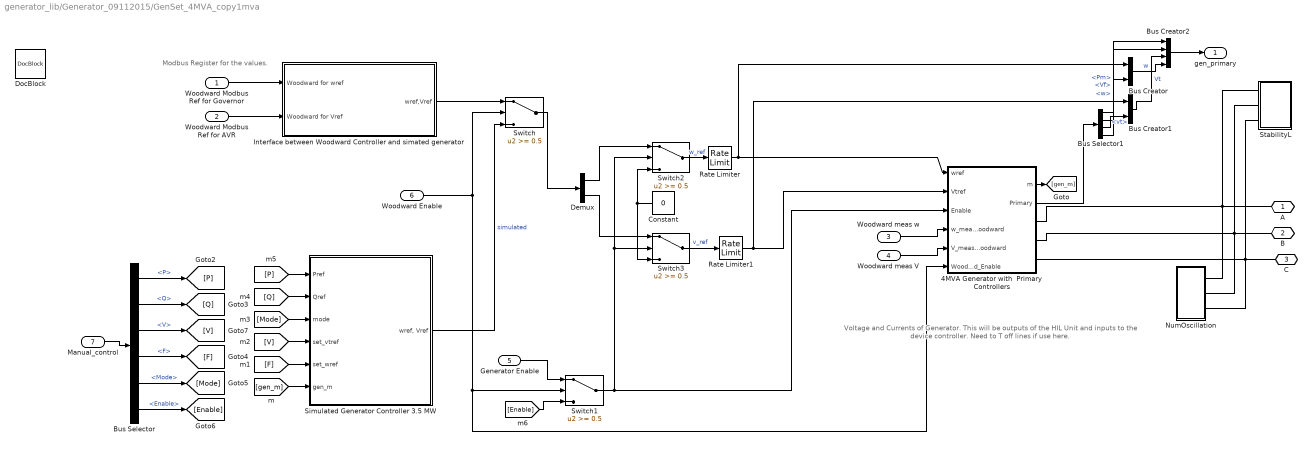
== system generator_lib/Generator_09112015/GenSet_4MVA_copy1mva ==
  note: Modbus Register for the values.
  note: Voltage and Currents of Generator.
      | This will be outputs of the HIL Unit
      | and inputs to the device controller.
      | Need to T off lines if use here.
  Woodward Modbus Ref for Governor : Inport
  Woodward Modbus Ref for AVR : Inport  Port=2
  Woodward meas w : Inport  Port=3
  Woodward meas V : Inport  Port=4
  Generator Enable : Inport  Port=5
  Woodward Enable : Inport  Port=6
  Manual_control : Inport  Port=7
  4MVA Generator with  Primary Controllers : Subsystem
  Bus Creator : BusCreator  Inputs=2
  Bus Creator1 : BusCreator  Inputs=2
  Bus Creator2 : BusCreator
  Bus Selector : BusSelector  OutputSignals=P,Q,V,F,Mode,Enable
  Bus Selector1 : BusSelector  OutputSignals=Pm,Vf,vt,w
  Constant : Constant  Value=0
  Demux : Demux  Outputs=2
  DocBlock : simulink/Model-Wide Utilities/DocBlock  DocumentType=Text
  Interface between Woodward Controller and simated generator : Subsystem
  NumOscillation : Subsystem
  Rate Limiter : RateLimiter  RisingSlewLimit=0.5  FallingSlewLimit=-0.5  SampleTimeMode=inherited
  Rate Limiter1 : RateLimiter  RisingSlewLimit=0.5  FallingSlewLimit=-0.5  SampleTimeMode=inherited
  Simulated Generator Controller 3.5 MW : Subsystem
  StabilityL : Subsystem  mask{v=13800, kVA=300, pf=1}
  Switch{,1..3} (4 alike) : Switch  Threshold=0.5
  A : PMIOPort  Port=1  Side=Right
  B : PMIOPort  Port=2  Side=Right
  C : PMIOPort  Port=3  Side=Right
  gen_primary : Outport
  wires:
  [F] -> Simulated Generator Controller 3.5 MW/5(set_wref)
  [V] -> Simulated Generator Controller 3.5 MW/4(set_vtref)
  [Mode] -> Simulated Generator Controller 3.5 MW/3(mode)
  [Q] -> Simulated Generator Controller 3.5 MW/2(Qref)
  [P] -> Simulated Generator Controller 3.5 MW/1(Pref)
  [gen_m] -> Simulated Generator Controller 3.5 MW/6(gen_m)
  Bus Selector/5 -> [Mode]  "<Mode>"
  Bus Selector/4 -> [F]  "<F>"
  Bus Selector/3 -> [V]  "<V>"
  Bus Selector/2 -> [Q]  "<Q>"
  Bus Selector/1 -> [P]  "<P>"
  Manual_control/1 -> Bus Selector/1
  Simulated Generator Controller 3.5 MW/1("wref, Vref") -> Switch/3  "simulated"
  4MVA Generator with  Primary Controllers/1(m) -> [gen_m]
  Interface between Woodward Controller and simated generator/1(wref,Vref) -> Switch/1
  Switch/1 -> Demux/1
  Woodward Modbus Ref for Governor/1 -> Interface between Woodward Controller and simated generator/1(Woodward for wref)
  Woodward Modbus Ref for AVR/1 -> Interface between Woodward Controller and simated generator/2(Woodward for Vref)
  Woodward meas w/1 -> 4MVA Generator with  Primary Controllers/4(w_meas_Woodward)
  Woodward meas V/1 -> 4MVA Generator with  Primary Controllers/5(V_meas_Woodward)
  Bus Selector/6 -> [Enable]  "<Enable>"
  4MVA Generator with  Primary Controllers/2(Primary) -> Bus Selector1/1
  Generator Enable/1 -> Switch1/1
  [Enable] -> Switch1/3
  Switch1/1 -> 4MVA Generator with  Primary Controllers/3(Enable), Switch2/2, Switch3/2
  Switch2/1 -> Rate Limiter/1  "w_ref"
  Demux/1 -> Switch2/1
  Demux/2 -> Switch3/1
  Constant/1 -> Switch3/3, Switch2/3
  Switch3/1 -> Rate Limiter1/1  "v_ref"
  Bus Selector1/3 -> Bus Creator1/2  "<vt>"
  Bus Selector1/4 -> Bus Creator/2  "<w>"
  Bus Selector1/2 -> Bus Creator2/2  "<Vf>"
  Bus Selector1/1 -> Bus Creator2/1  "<Pm>"
  Bus Creator1/1 -> Bus Creator2/3  "Vt"
  Bus Creator/1 -> Bus Creator2/4  "w"
  Bus Creator2/1 -> gen_primary/1
  Rate Limiter/1 -> 4MVA Generator with  Primary Controllers/1(wref), Bus Creator/1
  Rate Limiter1/1 -> 4MVA Generator with  Primary Controllers/2(Vtref), Bus Creator1/1
  Woodward Enable/1 -> Switch/2, Switch1/2, 4MVA Generator with  Primary Controllers/6(Woodward_Enable)
  connections:
  StabilityL/LConn1 -- A/RConn1 -- 4MVA Generator with  Primary Controllers/RConn1 -- NumOscillation/LConn1
  StabilityL/LConn2 -- 4MVA Generator with  Primary Controllers/RConn2 -- B/RConn1 -- NumOscillation/LConn2
  StabilityL/LConn3 -- C/RConn1 -- 4MVA Generator with  Primary Controllers/RConn3 -- NumOscillation/LConn3

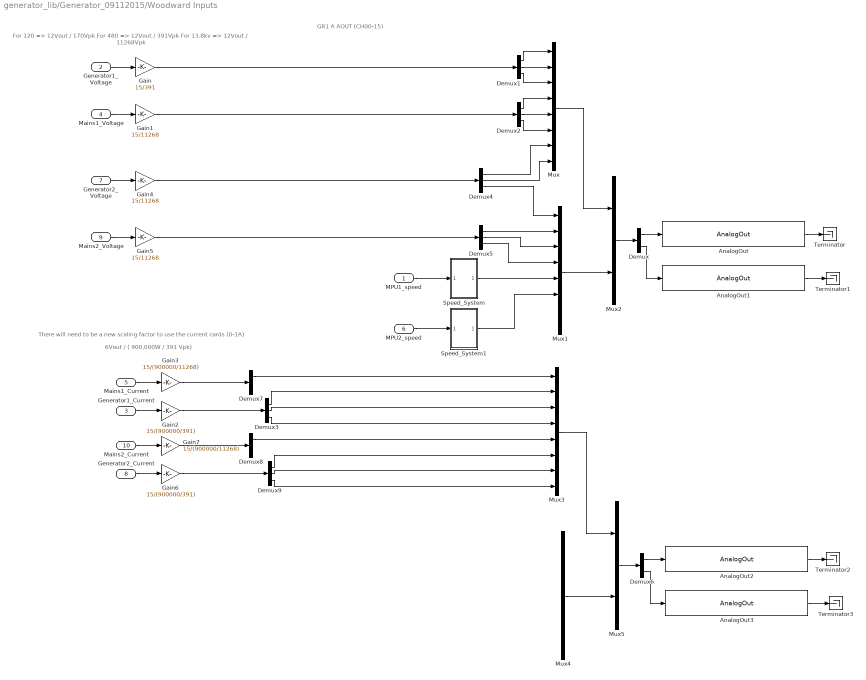
== system generator_lib/Generator_09112015/Woodward Inputs ==
  note: 6Vout / ( 900,000W / 391 Vpk)
  note: For 120 => 12Vout / 170Vpk
      | For 480 => 12Vout / 391Vpk
      | For 13.8kv => 12Vout / 11268Vpk
  note: GR1 A AOUT (CH00-15)
  note: There will need to be a
      | new scaling factor to use
      | the current cards (0-1A)
  MPU1_speed : Inport
  Generator1_Voltage : Inport  Port=2
  Generator1_Current : Inport  Port=3
  Mains1_Voltage : Inport  Port=4
  Mains1_Current : Inport  Port=5
  MPU2_speed : Inport  Port=6
  Generator2_Voltage : Inport  Port=7
  Generator2_Current : Inport  Port=8
  Mains2_Voltage : Inport  Port=9
  Mains2_Current : Inport  Port=10
  AnalogOut : rtio_opalrt_common/AnalogOut  CtrlName='OpCtrl'  portNb=1  FcnNos=Slot 1 Module A Subsection 1  size=16  maxcount=-2  count=8  numchan=8  israngeinput=off  voltagerange=[-16 ... 16]  slot=0  side=0  mismatch=0  slotside=Slot_1_Module_A
      settings: AttributesFormatString=%<CtrlName>
  AnalogOut1 : rtio_opalrt_common/AnalogOut  CtrlName='OpCtrl'  portNb=2  FcnNos=Slot 1 Module A Subsection 2  size=16  maxcount=-2  count=8  numchan=8  israngeinput=off  voltagerange=[-16 ... 16]  slot=0  side=0  mismatch=0  slotside=Slot_1_Module_A
      settings: AttributesFormatString=%<CtrlName>
  AnalogOut2 : rtio_opalrt_common/AnalogOut  CtrlName='OpCtrl'  portNb=3  FcnNos=Slot 2 Module A Subsection 1  size=16  maxcount=-2  count=8  numchan=8  israngeinput=off  voltagerange=[-16 ... 16]  slot=1  side=0  mismatch=0  slotside=Slot_2_Module_A
      settings: AttributesFormatString=%<CtrlName>
  AnalogOut3 : rtio_opalrt_common/AnalogOut  CtrlName='OpCtrl'  portNb=4  FcnNos=Slot 2 Module A Subsection 2  size=16  maxcount=-2  count=8  numchan=8  israngeinput=off  voltagerange=[-16 ... 16]  slot=1  side=0  mismatch=0  slotside=Slot_2_Module_A
      settings: AttributesFormatString=%<CtrlName>
  Demux : Demux  Outputs=2
  Demux{1..5,7..9} (8 alike) : Demux  Outputs=3
  Demux6 : Demux  Outputs=2
  Gain : Gain  Gain=15/391
  Gain1 : Gain  Gain=15/11268
  Gain2 : Gain  Gain=15/(900000/391)
  Gain3 : Gain  Gain=15/(900000/11268)
  Gain4 : Gain  Gain=15/11268
  Gain5 : Gain  Gain=15/11268
  Gain6 : Gain  Gain=15/(900000/391)
  Gain7 : Gain  Gain=15/(900000/11268)
  Mux{,1,3..4} (4 alike) : Mux  Inputs=8
  Mux2 : Mux  Inputs=2
  Mux5 : Mux  Inputs=2
  Speed_System : Subsystem
  Speed_System1 : Subsystem
  Terminator{,1..3} (4 alike) : Terminator
  wires:
  MPU1_speed/1 -> Speed_System/1(In1)
  Generator1_Current/1 -> Gain2/1
  Gain1/1 -> Demux2/1
  Gain/1 -> Demux1/1
  Mains1_Voltage/1 -> Gain1/1
  Mux2/1 -> Demux/1
  Mux1/1 -> Mux2/2
  Mux/1 -> Mux2/1
  Generator1_Voltage/1 -> Gain/1
  Demux/2 -> AnalogOut1/1
  Demux/1 -> AnalogOut/1
  AnalogOut1/1 -> Terminator1/1
  AnalogOut/1 -> Terminator/1
  Demux1/1 -> Mux/1
  Demux1/2 -> Mux/2
  Demux1/3 -> Mux/3
  Demux2/1 -> Mux/4
  Demux2/2 -> Mux/5
  Demux2/3 -> Mux/6
  Speed_System/1(Out1) -> Mux1/5
  Demux4/1 -> Mux/7
  Demux4/2 -> Mux/8
  Demux4/3 -> Mux1/1
  Demux5/1 -> Mux1/2
  Demux5/2 -> Mux1/3
  Demux5/3 -> Mux1/4
  Mux5/1 -> Demux6/1
  Mux4/1 -> Mux5/2
  Mux3/1 -> Mux5/1
  Demux6/2 -> AnalogOut3/1
  Demux6/1 -> AnalogOut2/1
  AnalogOut3/1 -> Terminator3/1
  AnalogOut2/1 -> Terminator2/1
  Gain2/1 -> Demux3/1
  Demux3/1 -> Mux3/2
  Demux3/2 -> Mux3/3
  Demux3/3 -> Mux3/4
  Mains1_Current/1 -> Gain3/1
  Gain3/1 -> Demux7/1
  Demux7/1 -> Mux3/1
  Gain5/1 -> Demux5/1
  Gain4/1 -> Demux4/1
  Mains2_Voltage/1 -> Gain5/1
  Generator2_Voltage/1 -> Gain4/1
  MPU2_speed/1 -> Speed_System1/1(In1)
  Speed_System1/1(Out1) -> Mux1/6
  Generator2_Current/1 -> Gain6/1
  Mains2_Current/1 -> Gain7/1
  Gain7/1 -> Demux8/1
  Demux8/1 -> Mux3/5
  Gain6/1 -> Demux9/1
  Demux9/1 -> Mux3/6
  Demux9/2 -> Mux3/7
  Demux9/3 -> Mux3/8

== system generator_lib/Generator_09112015/Woodward Outputs ==
  Digital Output : Inport
  DIO Enable : Inport  Port=2
  Bias Enable : Inport  Port=3
  Bus Creator1 : BusCreator  Inputs=3
  DIO - Gr3 : Subsystem
  DIO - Woodward : Subsystem
  DOUT type config : Subsystem
  OpCtrl : rtio_opalrt_common/OpCtrl  CtrlName='OpCtrl'  boardid=0  BitstreamFilename=VC707_2-EX-0001-2_2_6_61-32AIO16DIO16DIOSel-01-01.bin  numconfig=-1  mode=Master  externalClock=off  decimRtsi=0  calibIO=off  SampleTime=0  loadinport=-1  BoardType=VC707  SecondaryPresent=off  sync_type=Audio
  PWM IO - Gr3 : Subsystem
  TSDIO - Gr3 : Subsystem
  Woodward Primary Inputs : Subsystem
  Error : Outport
  IDs : Outport  Port=2
  Digital Inputs : Outport  Port=3
  Gen1 Gov and AVR : Outport  Port=4
  Gen2 Gov and AVR : Outport  Port=5
  Gen1 Fuel Enable : Outport  Port=6
  Gen1 GCB : Outport  Port=7
  Gen1 MCB : Outport  Port=8
  Gen2 Fuel Enable : Outport  Port=9
  Gen2 GCB : Outport  Port=10
  Gen2 MCB : Outport  Port=11
  wires:
  OpCtrl/1 -> Error/1
  OpCtrl/2 -> IDs/1
  DIO - Woodward/4(DIn1) -> DIO - Gr3/1(Dout)
  PWM IO - Gr3/1(PWMIn) -> Bus Creator1/3  "PWMIN"
  TSDIO - Gr3/1(TSDin) -> Bus Creator1/2  "TSDIN"
  DIO - Gr3/1(DIn) -> Bus Creator1/1, DIO - Woodward/1(Din_Wood1)  "DIN"
  Bus Creator1/1 -> Digital Inputs/1
  DIO Enable/1 -> DIO - Woodward/3(control), DIO - Woodward/4(control1)
  Woodward Primary Inputs/1(Gen1 Gov and AVR) -> Gen1 Gov and AVR/1
  Woodward Primary Inputs/2(Gen2 Gov and AVR) -> Gen2 Gov and AVR/1
  Bias Enable/1 -> Woodward Primary Inputs/1(Bias-ctrl)
  Digital Output/1 -> DIO - Woodward/2(Din_sim), PWM IO - Gr3/1(PWMOut), TSDIO - Gr3/1(TSDout)
  DIO - Woodward/2(Gen1 GCB) -> Gen1 GCB/1
  DIO - Woodward/3(Gen1 MCB) -> Gen1 MCB/1
  DIO - Woodward/1(Gen1 Fuel Enable) -> Gen1 Fuel Enable/1
  DIO - Woodward/6(Gen2 GCB) -> Gen2 GCB/1
  DIO - Woodward/5(Gen2 Fuel Enable) -> Gen2 Fuel Enable/1
  DIO - Woodward/7(Gen2 MCB) -> Gen2 MCB/1
